simulink model "EMI_Resilient_Actuator_Phase2B"  (R2026a)
settings: Solver=FixedStepDiscrete  StopTime=1.5  FixedStep=0.001
settings Model: Creator=adand  LastModifiedBy=adand

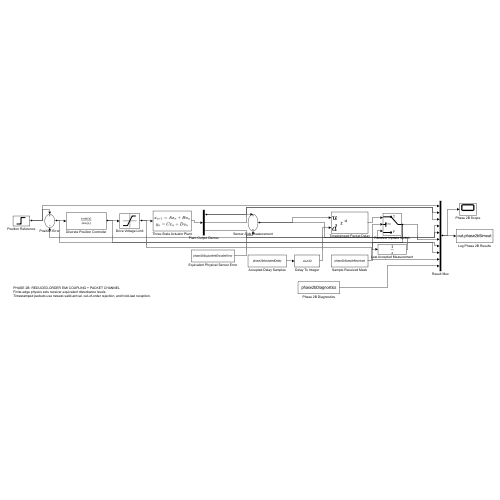
[thumbnail: Simulink's stored preview of the top-level diagram]
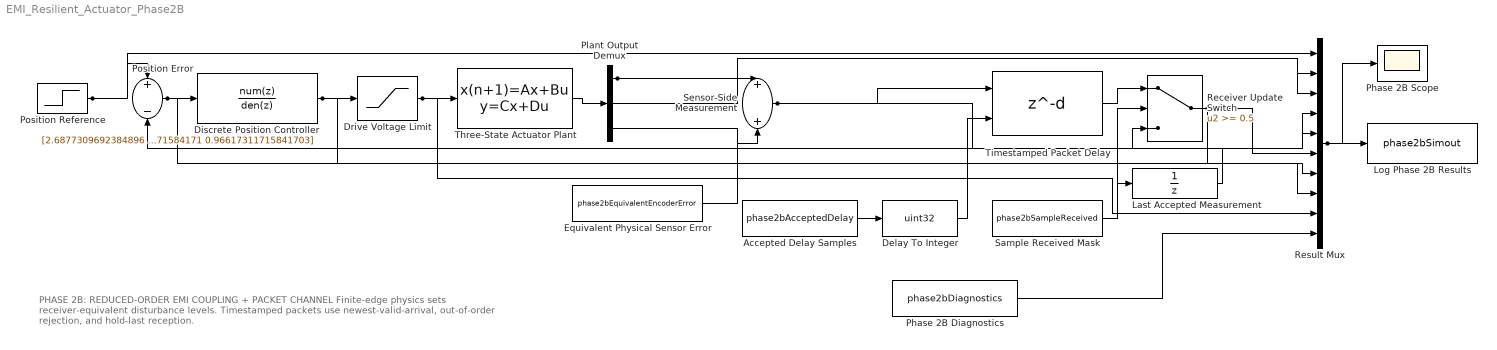
== system EMI_Resilient_Actuator_Phase2B ==
  note: PHASE 2B: REDUCED-ORDER EMI COUPLING + PACKET CHANNEL
      | Finite-edge physics sets receiver-equivalent disturbance levels.
      | Timestamped packets use newest-valid-arrival, out-of-order rejection, and hold-last reception.
  Accepted Delay Samples : FromWorkspace  VariableName=phase2bAcceptedDelay  Interpolate=off  OutputAfterFinalValue=Holding final value
  Delay To Integer : DataTypeConversion  OutDataTypeStr=uint32  SaturateOnIntegerOverflow=off  RndMeth=Floor
  Discrete Position Controller : DiscreteTransferFcn  Numerator=[2.6877309692384896 -5.3193946526740499 2.6318328983800279]  Denominator=[1 -1.9661731171584171 0.96617311715841703]  SampleTime=0.001
  Drive Voltage Limit : Saturate  UpperLimit=24  LowerLimit=-24
  Equivalent Physical Sensor Error : FromWorkspace  VariableName=phase2bEquivalentEncoderError  Interpolate=off  OutputAfterFinalValue=Holding final value
  Last Accepted Measurement : UnitDelay  SampleTime=0.001
  Log Phase 2B Results : ToWorkspace  VariableName=phase2bSimout  SaveFormat=Structure With Time  SampleTime=-1
  Phase 2B Diagnostics : FromWorkspace  VariableName=phase2bDiagnostics  Interpolate=off  OutputAfterFinalValue=Holding final value
  Phase 2B Scope : Scope
  Plant Output Demux : Demux  Outputs=3
  Position Error : Sum  Inputs=+-
  Position Reference : Step  Time=0.10000000000000001  FinalValue=0.52359877559829882  SampleTime=0.001
  Receiver Update Switch : Switch  Threshold=0.5  SaturateOnIntegerOverflow=off  InputSameDT=off
  Result Mux : Mux  Inputs=10
  Sample Received Mask : FromWorkspace  VariableName=phase2bSampleReceived  Interpolate=off  OutputAfterFinalValue=Holding final value
  Sensor-Side Measurement : Sum
  Three-State Actuator Plant : DiscreteStateSpace  A=[1 0.0009971362516155032 0.00022829831371848575;0 0.99202969645993144 0.42222281027672853;0 -0.025333368616603714 0.61255694572372166]  B=[3.1636509108574085e-05;0.09131932548739434;0.31678125686440572]  C=[1 0 0;0 1 0;0 0 1]  D=[0;0;0]  InitialCondition=zeros(3,1)  SampleTime=0.001
  Timestamped Packet Delay : Delay  DelayLengthSource=Input port  DelayLengthUpperLimit=16  InitialCondition=0  DiagnosticForDelayLength=Error  SampleTime=0.001
      settings: InputPortMap=u0,p1
  wires:
  Position Reference/1 -> Position Error/1, Result Mux/1
  Position Error/1 -> Discrete Position Controller/1, Result Mux/7
  Discrete Position Controller/1 -> Drive Voltage Limit/1, Result Mux/8
  Drive Voltage Limit/1 -> Three-State Actuator Plant/1, Result Mux/9
  Three-State Actuator Plant/1 -> Plant Output Demux/1
  Plant Output Demux/1 -> Sensor-Side Measurement/1, Result Mux/2
  Equivalent Physical Sensor Error/1 -> Sensor-Side Measurement/2
  Sensor-Side Measurement/1 -> Timestamped Packet Delay/1, Result Mux/5
  Accepted Delay Samples/1 -> Delay To Integer/1
  Delay To Integer/1 -> Timestamped Packet Delay/2
  Timestamped Packet Delay/1 -> Receiver Update Switch/1
  Sample Received Mask/1 -> Receiver Update Switch/2
  Last Accepted Measurement/1 -> Receiver Update Switch/3
  Receiver Update Switch/1 -> Last Accepted Measurement/1, Position Error/2, Result Mux/6
  Plant Output Demux/2 -> Result Mux/3
  Plant Output Demux/3 -> Result Mux/4
  Phase 2B Diagnostics/1 -> Result Mux/10
  Result Mux/1 -> Phase 2B Scope/1, Log Phase 2B Results/1
